simulink model "Impcont_foot_test2"  (R2016a)
settings: Solver=ode23tb  StartTime=0.0  StopTime=ti(end)  MaxStep=1e-3
InitFcn:
  | fp_sp_k = 12e3;
  | fp_sp_d = 1;
  | weights = 70/6;
  | joint_k = 0*180/pi;
  | joint_d = 0*180/pi;
  | fp_uj_dp_k = 500*180/pi;
  | fp_uj_dp_d = 1*180/pi;
  | fp_uj_ie_k = 500*180/pi;
  | fp_uj_ie_d = 1*180/pi;
  | 
  | x_k = 0*180/pi; x_d = 0*180/pi;
  | y_k = 0*180/pi; y_d = 0*180/pi;
  | z_k = 0*180/pi; z_d = 0*180/pi;
  | 
  | %{
  | stiff_dp=0.1*180/pi; stiff_ie=1*180/pi;
  | damp_dp=1*180/pi; damp_ie=1*180/pi;
  | % offset of prosthesis from centre of FP (XZY)
  |  sta=[-0.5345-6.54e-2 0.03779 0];
  | %}
  | 
  | % initpos = inv(jacob_gaitEmul(zeros(6,1)))*[ankle.trans(1,:).'; zeros(3,1)];
  | 
  | % sta = -[initpos(1) initpos(2) initpos(3)];
StopFcn:
  | %{
  | ankle = struct('ang_dp', angle_dp_out.signals.values,'ang_ie', angle_ie_out.signals.values,...
  |            'vel_dp',vel_dp.signals.values,'vel_ie',vel_ie.signals.values,...
  |            'acc_dp',acc_dp.signals.values,'acc_ie',acc_ie.signals.values,...
  |            'trans',ankle_trans_out.signals.values);
  | shin = struct('trans', trans_shin.signals.values, 'quat', quat_shin.signals.values);
  | foot = struct('trans', trans_foot.signals.values, 'quat', quat_foot.signals.values,...
  |     'acc',acc_foot.signals.values);
  | fplate = struct('trans', trans_fp.signals.values, 'quat', quat_fp.signals.values,...
  |     'torques', fp_torque_out.signals.values, 'forces', fp_force_out.signals.values);
  | 
  | [~, ~, ankle_ej.trans, ~] = est_joint(shin, foot);
  | 
  | fpForce = quatrotate(quatinv(fplate.quat), fplate.forces);
  | fpTorque = quatrotate(quatinv(fplate.quat), fplate.torques);
  | 
  | torque = cross(fplate.trans - ankle_ej.trans, fpForce) + fpTorque;
  | 
  | regMdl_dp = regress(torque(:,3),[ankle.ang_dp ankle.vel_dp foot.acc(:,3)]);
  | regMdl_ie = regress(torque(:,1),[ankle.ang_ie ankle.vel_ie foot.acc(:,1)]);
  | analysis_si = struct('kdp',regMdl_dp(1),'bdp',regMdl_dp(2),...
  |     'kie',regMdl_ie(1),'bie',regMdl_ie(2),'Jdp',regMdl_dp(3),...
  |     'Jie',regMdl_ie(3));
  | 
  | % %{
  | regMdl_dp = regress(torque(:,3),[ankle.ang_dp ankle.vel_dp ankle.acc_dp]);
  | regMdl_ie = regress(torque(:,1),[ankle.ang_ie ankle.vel_ie ankle.acc_ie]);
  | analysis_si2 = struct('kdp',regMdl_dp(1),'bdp',regMdl_dp(2),...
  |     'kie',regMdl_ie(1),'bie',regMdl_ie(2),'Jdp',regMdl_dp(3),...
  |     'Jie',regMdl_ie(3));
  | % %}
  | 
  | % %{
  | regMdl_dp = regress(tt_dp.signals.values(:,3),[ankle.ang_dp ankle.vel_dp ankle.acc_dp]);
  | regMdl_ie = regress(tt_ie.signals.values(:,3),[ankle.ang_ie ankle.vel_ie ankle.acc_ie]);
  | analysis_si3 = struct('kdp',regMdl_dp(1),'bdp',regMdl_dp(2),...
  |     'kie',regMdl_ie(1),'bie',regMdl_ie(2),'Jdp',regMdl_dp(3),...
  |     'Jie',regMdl_ie(3));
  | % %}
  | 
  | % %{
  | regMdl_dp = regress(tt_dp.signals.values(:,3),[ankle.ang_dp ankle.vel_dp foot.acc(:,3)]);
  | regMdl_ie = regress(tt_ie.signals.values(:,3),[ankle.ang_ie ankle.vel_ie foot.acc(:,1)]);
  | analysis_si4 = struct('kdp',regMdl_dp(1),'bdp',regMdl_dp(2),...
  |     'kie',regMdl_ie(1),'bie',regMdl_ie(2),'Jdp',regMdl_dp(3),...
  |     'Jie',regMdl_ie(3));
  | % %}
  | 
  | regMdl_dp = regress(torque(:,3),[ankle.ang_dp ankle.vel_dp]);
  | regMdl_ie = regress(torque(:,1),[ankle.ang_ie ankle.vel_ie]);
  | analysis_si5 = struct('kdp',regMdl_dp(1),'bdp',regMdl_dp(2),...
  |     'kie',regMdl_ie(1),'bie',regMdl_ie(2));
  | 
  | %}
values from neighbouring files (symbols this model uses):
  N = length(shin_angles_in.signals.values)    [GaitEmu_code.m]    (also in dy1.m; dy2.m; est_joint.m = size( [body1.trans body2.trans], 1 ); impcont.m)
  s = [-atan((t2.*3.379e-4+t3+t4.*t5.*4.401e-2)./(t4.*cos(q2)));-asin(t2.*1.4870979e-5+t3.*4.401e-2-t4.*t5)]    [FK_af.m]    (also in FK_footimp.m = [atan((ree2_1.*t2.*4.401e-2+ree2_2.*t4+ree2_3.*t3+t5.*t7.*4.; FK_gaitEmul.m = [q1+t2.*t4.*4.234e-1+t3.*t5.*1.5e-3-t2.*t6.*t7.*1.5e-3-5.347; ik.m = [x; y; z]; ik_af.m = FK_af(q))
  Y = -( reshape( body1.trans', [], 1 ) - reshape( body2.trans', [], 1 ) )    [creat_joint.m]    (also in est_joint.m = -( reshape( body1.trans', [3*N 1] ) - reshape( body2.trans',)
undefined symbols (not defined in the file or in its folder): X, Z
libraries: sm_lib x274, nesl_utility x97, simulink x3, dspstat3 x2, aerolibtransform2 x1
(part 7 of 7)

== system Impcont_foot_test2/Gait Emulator/prismatic frame1/y_bar_w_weightWalk_Sim1_1_RIGID/weight_4_RIGID ==
  ReferenceFrame : sm_lib/Frames and Transforms/Reference Frame
  Solid : sm_lib/Body Elements/Solid  InertiaType=Custom  Mass=weights  MassUnits=kg  CenterOfMass=[-0.093540130299891208 0.042272178743630776 0.014999999999999999]  CenterOfMassUnits=m  MomentsOfInertia=[0.0088271162208858108 0.0088271162208858108 0.017393538113134353]  MomentsOfInertiaUnits=kg*m^2  ProductsOfInertia=[0 0 0]  ProductsOfInertiaUnits=kg*m^2  DensityBased=on  Density=1000  DensityUnits=kg/(m^3)  DoExposeReferenceFrame=on  SerializedFrames=<Frames/>  GraphicType=FromGeometry  MarkerShape=Sphere  MarkerSize=10  MarkerSizeUnits=m  GraphicVisPropType=SimpleVisualProperties  GraphicDiffuseColor=[0.792156862745098 0.81960784313725488 0.93333333333333335]  GraphicSpecularColor=[0.5 0.5 0.5 1.0]  GraphicAmbientColor=[0.15 0.15 0.15 1.0]  GraphicEmissiveColor=[0.0 0.0 0.0 1.0]  GraphicShininess=75  GraphicOpacity=1  GeometryShape=FromFile  RectangleSize=[1 1]  RectangleSizeUnits=m  BrickDimensions=[1 1 1]  BrickDimensionUnits=m  CylinderRadius=1  CylinderRadiusUnits=m  CylinderLength=1  CylinderLengthUnits=m  SphereRadius=1  SphereRadiusUnits=m  EllipsoidRadii=[1 1 1]  EllipsoidRadiiUnits=m  ExtrusionCrossSection=[1 1; -1 1; -1 -1; 1 -1]  ExtrusionCrossSectionUnits=m  ExtrusionLength=1  ExtrusionLengthUnits=m  PolygonNumSides=3  PolygonOuterRadius=1  PolygonOuterRadiusUnits=m  ExtGeomFileType=STL  ExtGeomFileName=weight_Default_sldprt.STL  ExtGeomFileUnits=m  RevolutionCrossSection=[1 1; 1 -1; 2 -1; 2 1]  RevolutionCrossSectionUnits=m  RevolutionExtent=Full  RevolutionAngle=180  RevolutionAngleUnits=deg
  F : PMIOPort  Port=1  Side=Left
  connections:
  Solid/RConn1 -- ReferenceFrame/RConn1 -- F/RConn1

== system Impcont_foot_test2/Gait Emulator/prismatic frame1/y_bar_w_weightWalk_Sim1_1_RIGID/weight_5_RIGID ==
  ReferenceFrame : sm_lib/Frames and Transforms/Reference Frame
  Solid : sm_lib/Body Elements/Solid  InertiaType=Custom  Mass=weights  MassUnits=kg  CenterOfMass=[-0.093540130299891208 0.042272178743630776 0.014999999999999999]  CenterOfMassUnits=m  MomentsOfInertia=[0.0088271162208858108 0.0088271162208858108 0.017393538113134353]  MomentsOfInertiaUnits=kg*m^2  ProductsOfInertia=[0 0 0]  ProductsOfInertiaUnits=kg*m^2  DensityBased=on  Density=1000  DensityUnits=kg/(m^3)  DoExposeReferenceFrame=on  SerializedFrames=<Frames/>  GraphicType=FromGeometry  MarkerShape=Sphere  MarkerSize=10  MarkerSizeUnits=m  GraphicVisPropType=SimpleVisualProperties  GraphicDiffuseColor=[0.792156862745098 0.81960784313725488 0.93333333333333335]  GraphicSpecularColor=[0.5 0.5 0.5 1.0]  GraphicAmbientColor=[0.15 0.15 0.15 1.0]  GraphicEmissiveColor=[0.0 0.0 0.0 1.0]  GraphicShininess=75  GraphicOpacity=1  GeometryShape=FromFile  RectangleSize=[1 1]  RectangleSizeUnits=m  BrickDimensions=[1 1 1]  BrickDimensionUnits=m  CylinderRadius=1  CylinderRadiusUnits=m  CylinderLength=1  CylinderLengthUnits=m  SphereRadius=1  SphereRadiusUnits=m  EllipsoidRadii=[1 1 1]  EllipsoidRadiiUnits=m  ExtrusionCrossSection=[1 1; -1 1; -1 -1; 1 -1]  ExtrusionCrossSectionUnits=m  ExtrusionLength=1  ExtrusionLengthUnits=m  PolygonNumSides=3  PolygonOuterRadius=1  PolygonOuterRadiusUnits=m  ExtGeomFileType=STL  ExtGeomFileName=weight_Default_sldprt.STL  ExtGeomFileUnits=m  RevolutionCrossSection=[1 1; 1 -1; 2 -1; 2 1]  RevolutionCrossSectionUnits=m  RevolutionExtent=Full  RevolutionAngle=180  RevolutionAngleUnits=deg
  F : PMIOPort  Port=1  Side=Left
  connections:
  Solid/RConn1 -- ReferenceFrame/RConn1 -- F/RConn1

== system Impcont_foot_test2/Gait Emulator/prismatic frame1/y_bar_w_weightWalk_Sim1_1_RIGID/weight_6_RIGID ==
  ReferenceFrame : sm_lib/Frames and Transforms/Reference Frame
  Solid : sm_lib/Body Elements/Solid  InertiaType=Custom  Mass=weights  MassUnits=kg  CenterOfMass=[-0.093540130299891208 0.042272178743630776 0.014999999999999999]  CenterOfMassUnits=m  MomentsOfInertia=[0.0088271162208858108 0.0088271162208858108 0.017393538113134353]  MomentsOfInertiaUnits=kg*m^2  ProductsOfInertia=[0 0 0]  ProductsOfInertiaUnits=kg*m^2  DensityBased=on  Density=1000  DensityUnits=kg/(m^3)  DoExposeReferenceFrame=on  SerializedFrames=<Frames/>  GraphicType=FromGeometry  MarkerShape=Sphere  MarkerSize=10  MarkerSizeUnits=m  GraphicVisPropType=SimpleVisualProperties  GraphicDiffuseColor=[0.792156862745098 0.81960784313725488 0.93333333333333335]  GraphicSpecularColor=[0.5 0.5 0.5 1.0]  GraphicAmbientColor=[0.15 0.15 0.15 1.0]  GraphicEmissiveColor=[0.0 0.0 0.0 1.0]  GraphicShininess=75  GraphicOpacity=1  GeometryShape=FromFile  RectangleSize=[1 1]  RectangleSizeUnits=m  BrickDimensions=[1 1 1]  BrickDimensionUnits=m  CylinderRadius=1  CylinderRadiusUnits=m  CylinderLength=1  CylinderLengthUnits=m  SphereRadius=1  SphereRadiusUnits=m  EllipsoidRadii=[1 1 1]  EllipsoidRadiiUnits=m  ExtrusionCrossSection=[1 1; -1 1; -1 -1; 1 -1]  ExtrusionCrossSectionUnits=m  ExtrusionLength=1  ExtrusionLengthUnits=m  PolygonNumSides=3  PolygonOuterRadius=1  PolygonOuterRadiusUnits=m  ExtGeomFileType=STL  ExtGeomFileName=weight_Default_sldprt.STL  ExtGeomFileUnits=m  RevolutionCrossSection=[1 1; 1 -1; 2 -1; 2 1]  RevolutionCrossSectionUnits=m  RevolutionExtent=Full  RevolutionAngle=180  RevolutionAngleUnits=deg
  F : PMIOPort  Port=1  Side=Left
  connections:
  Solid/RConn1 -- ReferenceFrame/RConn1 -- F/RConn1

== system Impcont_foot_test2/Gait Emulator/prismatic frame1/y_bar_w_weightWalk_Sim1_1_RIGID/y_bar_1_RIGID ==
  ReferenceFrame : sm_lib/Frames and Transforms/Reference Frame
  Solid : sm_lib/Body Elements/Solid  InertiaType=Custom  Mass=1.29  MassUnits=kg  CenterOfMass=[0.00076616175672379865 -0.25377093214757318 3.5664030409292288e-05]  CenterOfMassUnits=m  MomentsOfInertia=[0.010298158029361381 7.4602586681976561e-05 0.010304194450422657]*(0.1/0.47799554976271263)  MomentsOfInertiaUnits=kg*m^2  ProductsOfInertia=[-6.4284014840620861e-08 -2.8526588755049515e-07 -1.380997973988322e-06]*(0.1/0.47799554976271263)  ProductsOfInertiaUnits=kg*m^2  DensityBased=on  Density=1000  DensityUnits=kg/(m^3)  DoExposeReferenceFrame=on  SerializedFrames=<Frames/>  GraphicType=FromGeometry  MarkerShape=Sphere  MarkerSize=10  MarkerSizeUnits=m  GraphicVisPropType=SimpleVisualProperties  GraphicDiffuseColor=[1.0 0.0 0.2]  GraphicSpecularColor=[0.5 0.5 0.5 1.0]  GraphicAmbientColor=[0.15 0.15 0.15 1.0]  GraphicEmissiveColor=[0.0 0.0 0.0 1.0]  GraphicShininess=75  GraphicOpacity=1  GeometryShape=FromFile  RectangleSize=[1 1]  RectangleSizeUnits=m  BrickDimensions=[1 1 1]  BrickDimensionUnits=m  CylinderRadius=1  CylinderRadiusUnits=m  CylinderLength=1  CylinderLengthUnits=m  SphereRadius=1  SphereRadiusUnits=m  EllipsoidRadii=[1 1 1]  EllipsoidRadiiUnits=m  ExtrusionCrossSection=[1 1; -1 1; -1 -1; 1 -1]  ExtrusionCrossSectionUnits=m  ExtrusionLength=1  ExtrusionLengthUnits=m  PolygonNumSides=3  PolygonOuterRadius=1  PolygonOuterRadiusUnits=m  ExtGeomFileType=STL  ExtGeomFileName=y_bar_Default_sldprt.STL  ExtGeomFileUnits=m  RevolutionCrossSection=[1 1; 1 -1; 2 -1; 2 1]  RevolutionCrossSectionUnits=m  RevolutionExtent=Full  RevolutionAngle=180  RevolutionAngleUnits=deg
  F : PMIOPort  Port=1  Side=Left
  connections:
  Solid/RConn1 -- ReferenceFrame/RConn1 -- F/RConn1

== system Impcont_foot_test2/Gait Emulator/Walkway & force plate/Force Plate/base_frame_1_RIGID/x8020_1020_1020_X_50cm_1_RIGID ==
  ReferenceFrame : sm_lib/Frames and Transforms/Reference Frame
  Solid : sm_lib/Body Elements/Solid  InertiaType=Custom  Mass=0.25907382645160842  MassUnits=kg  CenterOfMass=[0 0 0]  CenterOfMassUnits=in  MomentsOfInertia=[8.3933307234335093 8.4665424365077708 0.12805533197749852]  MomentsOfInertiaUnits=kg*in^2  ProductsOfInertia=[0 0 0]  ProductsOfInertiaUnits=kg*in^2  DensityBased=on  Density=1000  DensityUnits=kg/(m^3)  DoExposeReferenceFrame=on  SerializedFrames=<Frames/>  GraphicType=FromGeometry  MarkerShape=Sphere  MarkerSize=10  MarkerSizeUnits=m  GraphicVisPropType=SimpleVisualProperties  GraphicDiffuseColor=[1 1 1]  GraphicSpecularColor=[0.5 0.5 0.5 1.0]  GraphicAmbientColor=[0.15 0.15 0.15 1.0]  GraphicEmissiveColor=[0.0 0.0 0.0 1.0]  GraphicShininess=75  GraphicOpacity=1  GeometryShape=FromFile  RectangleSize=[1 1]  RectangleSizeUnits=m  BrickDimensions=[1 1 1]  BrickDimensionUnits=m  CylinderRadius=1  CylinderRadiusUnits=m  CylinderLength=1  CylinderLengthUnits=m  SphereRadius=1  SphereRadiusUnits=m  EllipsoidRadii=[1 1 1]  EllipsoidRadiiUnits=m  ExtrusionCrossSection=[1 1; -1 1; -1 -1; 1 -1]  ExtrusionCrossSectionUnits=m  ExtrusionLength=1  ExtrusionLengthUnits=m  PolygonNumSides=3  PolygonOuterRadius=1  PolygonOuterRadiusUnits=m  ExtGeomFileType=STL  ExtGeomFileName=8020-1020-1020 X 50cm_Default_sldprt.STL  ExtGeomFileUnits=in  RevolutionCrossSection=[1 1; 1 -1; 2 -1; 2 1]  RevolutionCrossSectionUnits=m  RevolutionExtent=Full  RevolutionAngle=180  RevolutionAngleUnits=deg
  F : PMIOPort  Port=1  Side=Left
  connections:
  ReferenceFrame/RConn1 -- Solid/RConn1 -- F/RConn1

== system Impcont_foot_test2/Gait Emulator/Walkway & force plate/Force Plate/base_frame_1_RIGID/x8020_1020_1020_X_50cm_2_RIGID ==
  ReferenceFrame : sm_lib/Frames and Transforms/Reference Frame
  Solid : sm_lib/Body Elements/Solid  InertiaType=Custom  Mass=0.25907382645160842  MassUnits=kg  CenterOfMass=[0 0 0]  CenterOfMassUnits=in  MomentsOfInertia=[8.3933307234335093 8.4665424365077708 0.12805533197749852]  MomentsOfInertiaUnits=kg*in^2  ProductsOfInertia=[0 0 0]  ProductsOfInertiaUnits=kg*in^2  DensityBased=on  Density=1000  DensityUnits=kg/(m^3)  DoExposeReferenceFrame=on  SerializedFrames=<Frames/>  GraphicType=FromGeometry  MarkerShape=Sphere  MarkerSize=10  MarkerSizeUnits=m  GraphicVisPropType=SimpleVisualProperties  GraphicDiffuseColor=[1 1 1]  GraphicSpecularColor=[0.5 0.5 0.5 1.0]  GraphicAmbientColor=[0.15 0.15 0.15 1.0]  GraphicEmissiveColor=[0.0 0.0 0.0 1.0]  GraphicShininess=75  GraphicOpacity=1  GeometryShape=FromFile  RectangleSize=[1 1]  RectangleSizeUnits=m  BrickDimensions=[1 1 1]  BrickDimensionUnits=m  CylinderRadius=1  CylinderRadiusUnits=m  CylinderLength=1  CylinderLengthUnits=m  SphereRadius=1  SphereRadiusUnits=m  EllipsoidRadii=[1 1 1]  EllipsoidRadiiUnits=m  ExtrusionCrossSection=[1 1; -1 1; -1 -1; 1 -1]  ExtrusionCrossSectionUnits=m  ExtrusionLength=1  ExtrusionLengthUnits=m  PolygonNumSides=3  PolygonOuterRadius=1  PolygonOuterRadiusUnits=m  ExtGeomFileType=STL  ExtGeomFileName=8020-1020-1020 X 50cm_Default_sldprt.STL  ExtGeomFileUnits=in  RevolutionCrossSection=[1 1; 1 -1; 2 -1; 2 1]  RevolutionCrossSectionUnits=m  RevolutionExtent=Full  RevolutionAngle=180  RevolutionAngleUnits=deg
  F : PMIOPort  Port=1  Side=Left
  connections:
  ReferenceFrame/RConn1 -- Solid/RConn1 -- F/RConn1

== system Impcont_foot_test2/Gait Emulator/Walkway & force plate/Force Plate/base_frame_1_RIGID/x8020_1020_1020_X_7_81_1_RIGID ==
  ReferenceFrame : sm_lib/Frames and Transforms/Reference Frame
  Solid : sm_lib/Body Elements/Solid  InertiaType=Custom  Mass=0.10278722807147889  MassUnits=kg  CenterOfMass=[0 0 0]  CenterOfMassUnits=in  MomentsOfInertia=[0.53334790666301179 0.56239456549511713 0.050805798463005557]  MomentsOfInertiaUnits=kg*in^2  ProductsOfInertia=[0 0 0]  ProductsOfInertiaUnits=kg*in^2  DensityBased=on  Density=1000  DensityUnits=kg/(m^3)  DoExposeReferenceFrame=on  SerializedFrames=<Frames/>  GraphicType=FromGeometry  MarkerShape=Sphere  MarkerSize=10  MarkerSizeUnits=m  GraphicVisPropType=SimpleVisualProperties  GraphicDiffuseColor=[1 1 1]  GraphicSpecularColor=[0.5 0.5 0.5 1.0]  GraphicAmbientColor=[0.15 0.15 0.15 1.0]  GraphicEmissiveColor=[0.0 0.0 0.0 1.0]  GraphicShininess=75  GraphicOpacity=1  GeometryShape=FromFile  RectangleSize=[1 1]  RectangleSizeUnits=m  BrickDimensions=[1 1 1]  BrickDimensionUnits=m  CylinderRadius=1  CylinderRadiusUnits=m  CylinderLength=1  CylinderLengthUnits=m  SphereRadius=1  SphereRadiusUnits=m  EllipsoidRadii=[1 1 1]  EllipsoidRadiiUnits=m  ExtrusionCrossSection=[1 1; -1 1; -1 -1; 1 -1]  ExtrusionCrossSectionUnits=m  ExtrusionLength=1  ExtrusionLengthUnits=m  PolygonNumSides=3  PolygonOuterRadius=1  PolygonOuterRadiusUnits=m  ExtGeomFileType=STL  ExtGeomFileName=8020-1020-1020 X 7_81_Default_sldprt.STL  ExtGeomFileUnits=in  RevolutionCrossSection=[1 1; 1 -1; 2 -1; 2 1]  RevolutionCrossSectionUnits=m  RevolutionExtent=Full  RevolutionAngle=180  RevolutionAngleUnits=deg
  F : PMIOPort  Port=1  Side=Left
  connections:
  ReferenceFrame/RConn1 -- Solid/RConn1 -- F/RConn1

== system Impcont_foot_test2/Gait Emulator/Walkway & force plate/Force Plate/base_frame_1_RIGID/x8020_1020_1020_X_7_81_2_RIGID ==
  ReferenceFrame : sm_lib/Frames and Transforms/Reference Frame
  Solid : sm_lib/Body Elements/Solid  InertiaType=Custom  Mass=0.10278722807147889  MassUnits=kg  CenterOfMass=[0 0 0]  CenterOfMassUnits=in  MomentsOfInertia=[0.53334790666301179 0.56239456549511713 0.050805798463005557]  MomentsOfInertiaUnits=kg*in^2  ProductsOfInertia=[0 0 0]  ProductsOfInertiaUnits=kg*in^2  DensityBased=on  Density=1000  DensityUnits=kg/(m^3)  DoExposeReferenceFrame=on  SerializedFrames=<Frames/>  GraphicType=FromGeometry  MarkerShape=Sphere  MarkerSize=10  MarkerSizeUnits=m  GraphicVisPropType=SimpleVisualProperties  GraphicDiffuseColor=[1 1 1]  GraphicSpecularColor=[0.5 0.5 0.5 1.0]  GraphicAmbientColor=[0.15 0.15 0.15 1.0]  GraphicEmissiveColor=[0.0 0.0 0.0 1.0]  GraphicShininess=75  GraphicOpacity=1  GeometryShape=FromFile  RectangleSize=[1 1]  RectangleSizeUnits=m  BrickDimensions=[1 1 1]  BrickDimensionUnits=m  CylinderRadius=1  CylinderRadiusUnits=m  CylinderLength=1  CylinderLengthUnits=m  SphereRadius=1  SphereRadiusUnits=m  EllipsoidRadii=[1 1 1]  EllipsoidRadiiUnits=m  ExtrusionCrossSection=[1 1; -1 1; -1 -1; 1 -1]  ExtrusionCrossSectionUnits=m  ExtrusionLength=1  ExtrusionLengthUnits=m  PolygonNumSides=3  PolygonOuterRadius=1  PolygonOuterRadiusUnits=m  ExtGeomFileType=STL  ExtGeomFileName=8020-1020-1020 X 7_81_Default_sldprt.STL  ExtGeomFileUnits=in  RevolutionCrossSection=[1 1; 1 -1; 2 -1; 2 1]  RevolutionCrossSectionUnits=m  RevolutionExtent=Full  RevolutionAngle=180  RevolutionAngleUnits=deg
  F : PMIOPort  Port=1  Side=Left
  connections:
  ReferenceFrame/RConn1 -- Solid/RConn1 -- F/RConn1

== system Impcont_foot_test2/Gait Emulator/Walkway & force plate/Force Plate/base_frame_1_RIGID/x8020_1020_1020_X_7_81_3_RIGID ==
  ReferenceFrame : sm_lib/Frames and Transforms/Reference Frame
  Solid : sm_lib/Body Elements/Solid  InertiaType=Custom  Mass=0.10278722807147889  MassUnits=kg  CenterOfMass=[0 0 0]  CenterOfMassUnits=in  MomentsOfInertia=[0.53334790666301179 0.56239456549511713 0.050805798463005557]  MomentsOfInertiaUnits=kg*in^2  ProductsOfInertia=[0 0 0]  ProductsOfInertiaUnits=kg*in^2  DensityBased=on  Density=1000  DensityUnits=kg/(m^3)  DoExposeReferenceFrame=on  SerializedFrames=<Frames/>  GraphicType=FromGeometry  MarkerShape=Sphere  MarkerSize=10  MarkerSizeUnits=m  GraphicVisPropType=SimpleVisualProperties  GraphicDiffuseColor=[1 1 1]  GraphicSpecularColor=[0.5 0.5 0.5 1.0]  GraphicAmbientColor=[0.15 0.15 0.15 1.0]  GraphicEmissiveColor=[0.0 0.0 0.0 1.0]  GraphicShininess=75  GraphicOpacity=1  GeometryShape=FromFile  RectangleSize=[1 1]  RectangleSizeUnits=m  BrickDimensions=[1 1 1]  BrickDimensionUnits=m  CylinderRadius=1  CylinderRadiusUnits=m  CylinderLength=1  CylinderLengthUnits=m  SphereRadius=1  SphereRadiusUnits=m  EllipsoidRadii=[1 1 1]  EllipsoidRadiiUnits=m  ExtrusionCrossSection=[1 1; -1 1; -1 -1; 1 -1]  ExtrusionCrossSectionUnits=m  ExtrusionLength=1  ExtrusionLengthUnits=m  PolygonNumSides=3  PolygonOuterRadius=1  PolygonOuterRadiusUnits=m  ExtGeomFileType=STL  ExtGeomFileName=8020-1020-1020 X 7_81_Default_sldprt.STL  ExtGeomFileUnits=in  RevolutionCrossSection=[1 1; 1 -1; 2 -1; 2 1]  RevolutionCrossSectionUnits=m  RevolutionExtent=Full  RevolutionAngle=180  RevolutionAngleUnits=deg
  F : PMIOPort  Port=1  Side=Left
  connections:
  ReferenceFrame/RConn1 -- Solid/RConn1 -- F/RConn1

== system Impcont_foot_test2/Gait Emulator/Walkway & force plate/Force Plate/top_frame_1_RIGID/frame1_1_RIGID ==
  ReferenceFrame : sm_lib/Frames and Transforms/Reference Frame
  Transform : sm_lib/Frames and Transforms/Rigid Transform  TranslationMethod=Cartesian  TranslationLengthUnit=m  TranslationStandardAxis=+Z  TranslationStandardOffset=0  TranslationCartesianOffset=[0.099187000000000025 -1.27675647831893e-15 -0.24999950000000001]  TranslationROffset=0  TranslationROffsetUnits=m  TranslationZOffset=0  TranslationZOffsetUnits=m  TranslationThetaOffset=0  TranslationThetaOffsetUnits=deg  RotationMethod=None  RotationAngleUnits=deg  RotationStandardAxis=+Z  RotationAngle=0.0  RotationArbitraryAxis=[0 0 1]  FollAlignAxisA=+X  BaseAlignAxisA=+Y  FollAlignAxisB=+Y  BaseAlignAxisB=+Z  RotationSequenceAxes=FollowerAxes  RotationSequence=XYX  RotationSequenceAngles=[0 0 0]  RotationSequenceAnglesUnits=deg  RotationMatrix=[1 0 0; 0 1 0; 0 0 1]
  Transform1 : sm_lib/Frames and Transforms/Rigid Transform  TranslationMethod=Cartesian  TranslationLengthUnit=m  TranslationStandardAxis=+Z  TranslationStandardOffset=0  TranslationCartesianOffset=[0.22377399999999997 0 -0.47459899999999999]  TranslationROffset=0  TranslationROffsetUnits=m  TranslationZOffset=0  TranslationZOffsetUnits=m  TranslationThetaOffset=0  TranslationThetaOffsetUnits=deg  RotationMethod=ArbitraryAxis  RotationAngleUnits=rad  RotationStandardAxis=+Z  RotationAngle=1.5707963267948968  RotationArbitraryAxis=[2.10991883731723e-15 1 5.8442032848726394e-16]  FollAlignAxisA=+X  BaseAlignAxisA=+Y  FollAlignAxisB=+Y  BaseAlignAxisB=+Z  RotationSequenceAxes=FollowerAxes  RotationSequence=XYX  RotationSequenceAngles=[0 0 0]  RotationSequenceAnglesUnits=deg  RotationMatrix=[1 0 0; 0 1 0; 0 0 1]
  Transform2 : sm_lib/Frames and Transforms/Rigid Transform  TranslationMethod=Cartesian  TranslationLengthUnit=m  TranslationStandardAxis=+Z  TranslationStandardOffset=0  TranslationCartesianOffset=[0.34836099999999992 -2.400857290751901e-15 -0.24999950000000001]  TranslationROffset=0  TranslationROffsetUnits=m  TranslationZOffset=0  TranslationZOffsetUnits=m  TranslationThetaOffset=0  TranslationThetaOffsetUnits=deg  RotationMethod=ArbitraryAxis  RotationAngleUnits=rad  RotationStandardAxis=+Z  RotationAngle=3.1415926535897931  RotationArbitraryAxis=[1.2403272853234171e-15 1 -5.0658111711395872e-16]  FollAlignAxisA=+X  BaseAlignAxisA=+Y  FollAlignAxisB=+Y  BaseAlignAxisB=+Z  RotationSequenceAxes=FollowerAxes  RotationSequence=XYX  RotationSequenceAngles=[0 0 0]  RotationSequenceAnglesUnits=deg  RotationMatrix=[1 0 0; 0 1 0; 0 0 1]
  Transform3 : sm_lib/Frames and Transforms/Rigid Transform  TranslationMethod=Cartesian  TranslationLengthUnit=m  TranslationStandardAxis=+Z  TranslationStandardOffset=0  TranslationCartesianOffset=[0.22377399999999986 -1.3322676295501878e-15 -0.025400000000000061]  TranslationROffset=0  TranslationROffsetUnits=m  TranslationZOffset=0  TranslationZOffsetUnits=m  TranslationThetaOffset=0  TranslationThetaOffsetUnits=deg  RotationMethod=ArbitraryAxis  RotationAngleUnits=rad  RotationStandardAxis=+Z  RotationAngle=1.5707963267948968  RotationArbitraryAxis=[-4.7691944979696082e-15 -1 -6.6899476726480988e-16]  FollAlignAxisA=+X  BaseAlignAxisA=+Y  FollAlignAxisB=+Y  BaseAlignAxisB=+Z  RotationSequenceAxes=FollowerAxes  RotationSequence=XYX  RotationSequenceAngles=[0 0 0]  RotationSequenceAnglesUnits=deg  RotationMatrix=[1 0 0; 0 1 0; 0 0 1]
  Transform4 : sm_lib/Frames and Transforms/Rigid Transform  TranslationMethod=Cartesian  TranslationLengthUnit=m  TranslationStandardAxis=+Z  TranslationStandardOffset=0  TranslationCartesianOffset=[-0.24999899999999994 0.025400000000001838 -0.22377400000000008]  TranslationROffset=0  TranslationROffsetUnits=m  TranslationZOffset=0  TranslationZOffsetUnits=m  TranslationThetaOffset=0  TranslationThetaOffsetUnits=deg  RotationMethod=ArbitraryAxis  RotationAngleUnits=rad  RotationStandardAxis=+Z  RotationAngle=1.5707963267948968  RotationArbitraryAxis=[-3.5952694497400173e-15 -1 1.7432631046654889e-15]  FollAlignAxisA=+X  BaseAlignAxisA=+Y  FollAlignAxisB=+Y  BaseAlignAxisB=+Z  RotationSequenceAxes=FollowerAxes  RotationSequence=XYX  RotationSequenceAngles=[0 0 0]  RotationSequenceAnglesUnits=deg  RotationMatrix=[1 0 0; 0 1 0; 0 0 1]
  x8020_1020_1020_X_50cm_1_RIGID : Subsystem
  x8020_1020_1020_X_50cm_2_RIGID : Subsystem
  x8020_1020_1020_X_7_81_1_RIGID : Subsystem
  x8020_1020_1020_X_7_81_2_RIGID : Subsystem
  F : PMIOPort  Port=1  Side=Right
  connections:
  Transform/RConn1 -- x8020_1020_1020_X_50cm_1_RIGID/LConn1
  Transform1/RConn1 -- x8020_1020_1020_X_7_81_1_RIGID/LConn1
  Transform2/RConn1 -- x8020_1020_1020_X_50cm_2_RIGID/LConn1
  Transform3/RConn1 -- x8020_1020_1020_X_7_81_2_RIGID/LConn1
  ReferenceFrame/RConn1 -- Transform2/LConn1 -- Transform3/LConn1 -- Transform/LConn1 -- Transform1/LConn1 -- Transform4/RConn1
  Transform4/LConn1 -- F/RConn1

== system Impcont_foot_test2/Gait Emulator/Walkway & force plate/Force Plate/top_frame_1_RIGID/x8020_1020_1020_X_11_81_1_RIGID ==
  ReferenceFrame : sm_lib/Frames and Transforms/Reference Frame
  Solid : sm_lib/Body Elements/Solid  InertiaType=Custom  Mass=0.15543113489425955  MassUnits=kg  CenterOfMass=[0 0 0]  CenterOfMassUnits=in  MomentsOfInertia=[1.8230290687756983 1.8669523774577936 0.076826693962624301]  MomentsOfInertiaUnits=kg*in^2  ProductsOfInertia=[0 0 0]  ProductsOfInertiaUnits=kg*in^2  DensityBased=on  Density=1000  DensityUnits=kg/(m^3)  DoExposeReferenceFrame=on  SerializedFrames=<Frames/>  GraphicType=FromGeometry  MarkerShape=Sphere  MarkerSize=10  MarkerSizeUnits=m  GraphicVisPropType=SimpleVisualProperties  GraphicDiffuseColor=[1 1 1]  GraphicSpecularColor=[0.5 0.5 0.5 1.0]  GraphicAmbientColor=[0.15 0.15 0.15 1.0]  GraphicEmissiveColor=[0.0 0.0 0.0 1.0]  GraphicShininess=75  GraphicOpacity=1  GeometryShape=FromFile  RectangleSize=[1 1]  RectangleSizeUnits=m  BrickDimensions=[1 1 1]  BrickDimensionUnits=m  CylinderRadius=1  CylinderRadiusUnits=m  CylinderLength=1  CylinderLengthUnits=m  SphereRadius=1  SphereRadiusUnits=m  EllipsoidRadii=[1 1 1]  EllipsoidRadiiUnits=m  ExtrusionCrossSection=[1 1; -1 1; -1 -1; 1 -1]  ExtrusionCrossSectionUnits=m  ExtrusionLength=1  ExtrusionLengthUnits=m  PolygonNumSides=3  PolygonOuterRadius=1  PolygonOuterRadiusUnits=m  ExtGeomFileType=STL  ExtGeomFileName=8020-1020-1020 X 11_81_Default_sldprt.STL  ExtGeomFileUnits=in  RevolutionCrossSection=[1 1; 1 -1; 2 -1; 2 1]  RevolutionCrossSectionUnits=m  RevolutionExtent=Full  RevolutionAngle=180  RevolutionAngleUnits=deg
  F : PMIOPort  Port=1  Side=Left
  connections:
  ReferenceFrame/RConn1 -- Solid/RConn1 -- F/RConn1

== system Impcont_foot_test2/Gait Emulator/Walkway & force plate/Force Plate/top_frame_1_RIGID/frame1_1_RIGID/x8020_1020_1020_X_50cm_1_RIGID ==
  ReferenceFrame : sm_lib/Frames and Transforms/Reference Frame
  Solid : sm_lib/Body Elements/Solid  InertiaType=Custom  Mass=0.25907382645160842  MassUnits=kg  CenterOfMass=[0 0 0]  CenterOfMassUnits=in  MomentsOfInertia=[8.3933307234335093 8.4665424365077708 0.12805533197749852]  MomentsOfInertiaUnits=kg*in^2  ProductsOfInertia=[0 0 0]  ProductsOfInertiaUnits=kg*in^2  DensityBased=on  Density=1000  DensityUnits=kg/(m^3)  DoExposeReferenceFrame=on  SerializedFrames=<Frames/>  GraphicType=FromGeometry  MarkerShape=Sphere  MarkerSize=10  MarkerSizeUnits=m  GraphicVisPropType=SimpleVisualProperties  GraphicDiffuseColor=[1 1 1]  GraphicSpecularColor=[0.5 0.5 0.5 1.0]  GraphicAmbientColor=[0.15 0.15 0.15 1.0]  GraphicEmissiveColor=[0.0 0.0 0.0 1.0]  GraphicShininess=75  GraphicOpacity=1  GeometryShape=FromFile  RectangleSize=[1 1]  RectangleSizeUnits=m  BrickDimensions=[1 1 1]  BrickDimensionUnits=m  CylinderRadius=1  CylinderRadiusUnits=m  CylinderLength=1  CylinderLengthUnits=m  SphereRadius=1  SphereRadiusUnits=m  EllipsoidRadii=[1 1 1]  EllipsoidRadiiUnits=m  ExtrusionCrossSection=[1 1; -1 1; -1 -1; 1 -1]  ExtrusionCrossSectionUnits=m  ExtrusionLength=1  ExtrusionLengthUnits=m  PolygonNumSides=3  PolygonOuterRadius=1  PolygonOuterRadiusUnits=m  ExtGeomFileType=STL  ExtGeomFileName=8020-1020-1020 X 50cm_Default_sldprt.STL  ExtGeomFileUnits=in  RevolutionCrossSection=[1 1; 1 -1; 2 -1; 2 1]  RevolutionCrossSectionUnits=m  RevolutionExtent=Full  RevolutionAngle=180  RevolutionAngleUnits=deg
  F : PMIOPort  Port=1  Side=Left
  connections:
  ReferenceFrame/RConn1 -- Solid/RConn1 -- F/RConn1

== system Impcont_foot_test2/Gait Emulator/Walkway & force plate/Force Plate/top_frame_1_RIGID/frame1_1_RIGID/x8020_1020_1020_X_50cm_2_RIGID ==
  ReferenceFrame : sm_lib/Frames and Transforms/Reference Frame
  Solid : sm_lib/Body Elements/Solid  InertiaType=Custom  Mass=0.25907382645160842  MassUnits=kg  CenterOfMass=[0 0 0]  CenterOfMassUnits=in  MomentsOfInertia=[8.3933307234335093 8.4665424365077708 0.12805533197749852]  MomentsOfInertiaUnits=kg*in^2  ProductsOfInertia=[0 0 0]  ProductsOfInertiaUnits=kg*in^2  DensityBased=on  Density=1000  DensityUnits=kg/(m^3)  DoExposeReferenceFrame=on  SerializedFrames=<Frames/>  GraphicType=FromGeometry  MarkerShape=Sphere  MarkerSize=10  MarkerSizeUnits=m  GraphicVisPropType=SimpleVisualProperties  GraphicDiffuseColor=[1 1 1]  GraphicSpecularColor=[0.5 0.5 0.5 1.0]  GraphicAmbientColor=[0.15 0.15 0.15 1.0]  GraphicEmissiveColor=[0.0 0.0 0.0 1.0]  GraphicShininess=75  GraphicOpacity=1  GeometryShape=FromFile  RectangleSize=[1 1]  RectangleSizeUnits=m  BrickDimensions=[1 1 1]  BrickDimensionUnits=m  CylinderRadius=1  CylinderRadiusUnits=m  CylinderLength=1  CylinderLengthUnits=m  SphereRadius=1  SphereRadiusUnits=m  EllipsoidRadii=[1 1 1]  EllipsoidRadiiUnits=m  ExtrusionCrossSection=[1 1; -1 1; -1 -1; 1 -1]  ExtrusionCrossSectionUnits=m  ExtrusionLength=1  ExtrusionLengthUnits=m  PolygonNumSides=3  PolygonOuterRadius=1  PolygonOuterRadiusUnits=m  ExtGeomFileType=STL  ExtGeomFileName=8020-1020-1020 X 50cm_Default_sldprt.STL  ExtGeomFileUnits=in  RevolutionCrossSection=[1 1; 1 -1; 2 -1; 2 1]  RevolutionCrossSectionUnits=m  RevolutionExtent=Full  RevolutionAngle=180  RevolutionAngleUnits=deg
  F : PMIOPort  Port=1  Side=Left
  connections:
  ReferenceFrame/RConn1 -- Solid/RConn1 -- F/RConn1

== system Impcont_foot_test2/Gait Emulator/Walkway & force plate/Force Plate/top_frame_1_RIGID/frame1_1_RIGID/x8020_1020_1020_X_7_81_1_RIGID ==
  ReferenceFrame : sm_lib/Frames and Transforms/Reference Frame
  Solid : sm_lib/Body Elements/Solid  InertiaType=Custom  Mass=0.10278722807147889  MassUnits=kg  CenterOfMass=[0 0 0]  CenterOfMassUnits=in  MomentsOfInertia=[0.53334790666301179 0.56239456549511713 0.050805798463005557]  MomentsOfInertiaUnits=kg*in^2  ProductsOfInertia=[0 0 0]  ProductsOfInertiaUnits=kg*in^2  DensityBased=on  Density=1000  DensityUnits=kg/(m^3)  DoExposeReferenceFrame=on  SerializedFrames=<Frames/>  GraphicType=FromGeometry  MarkerShape=Sphere  MarkerSize=10  MarkerSizeUnits=m  GraphicVisPropType=SimpleVisualProperties  GraphicDiffuseColor=[1 1 1]  GraphicSpecularColor=[0.5 0.5 0.5 1.0]  GraphicAmbientColor=[0.15 0.15 0.15 1.0]  GraphicEmissiveColor=[0.0 0.0 0.0 1.0]  GraphicShininess=75  GraphicOpacity=1  GeometryShape=FromFile  RectangleSize=[1 1]  RectangleSizeUnits=m  BrickDimensions=[1 1 1]  BrickDimensionUnits=m  CylinderRadius=1  CylinderRadiusUnits=m  CylinderLength=1  CylinderLengthUnits=m  SphereRadius=1  SphereRadiusUnits=m  EllipsoidRadii=[1 1 1]  EllipsoidRadiiUnits=m  ExtrusionCrossSection=[1 1; -1 1; -1 -1; 1 -1]  ExtrusionCrossSectionUnits=m  ExtrusionLength=1  ExtrusionLengthUnits=m  PolygonNumSides=3  PolygonOuterRadius=1  PolygonOuterRadiusUnits=m  ExtGeomFileType=STL  ExtGeomFileName=8020-1020-1020 X 7_81_Default_sldprt.STL  ExtGeomFileUnits=in  RevolutionCrossSection=[1 1; 1 -1; 2 -1; 2 1]  RevolutionCrossSectionUnits=m  RevolutionExtent=Full  RevolutionAngle=180  RevolutionAngleUnits=deg
  F : PMIOPort  Port=1  Side=Left
  connections:
  ReferenceFrame/RConn1 -- Solid/RConn1 -- F/RConn1

== system Impcont_foot_test2/Gait Emulator/Walkway & force plate/Force Plate/top_frame_1_RIGID/frame1_1_RIGID/x8020_1020_1020_X_7_81_2_RIGID ==
  ReferenceFrame : sm_lib/Frames and Transforms/Reference Frame
  Solid : sm_lib/Body Elements/Solid  InertiaType=Custom  Mass=0.10278722807147889  MassUnits=kg  CenterOfMass=[0 0 0]  CenterOfMassUnits=in  MomentsOfInertia=[0.53334790666301179 0.56239456549511713 0.050805798463005557]  MomentsOfInertiaUnits=kg*in^2  ProductsOfInertia=[0 0 0]  ProductsOfInertiaUnits=kg*in^2  DensityBased=on  Density=1000  DensityUnits=kg/(m^3)  DoExposeReferenceFrame=on  SerializedFrames=<Frames/>  GraphicType=FromGeometry  MarkerShape=Sphere  MarkerSize=10  MarkerSizeUnits=m  GraphicVisPropType=SimpleVisualProperties  GraphicDiffuseColor=[1 1 1]  GraphicSpecularColor=[0.5 0.5 0.5 1.0]  GraphicAmbientColor=[0.15 0.15 0.15 1.0]  GraphicEmissiveColor=[0.0 0.0 0.0 1.0]  GraphicShininess=75  GraphicOpacity=1  GeometryShape=FromFile  RectangleSize=[1 1]  RectangleSizeUnits=m  BrickDimensions=[1 1 1]  BrickDimensionUnits=m  CylinderRadius=1  CylinderRadiusUnits=m  CylinderLength=1  CylinderLengthUnits=m  SphereRadius=1  SphereRadiusUnits=m  EllipsoidRadii=[1 1 1]  EllipsoidRadiiUnits=m  ExtrusionCrossSection=[1 1; -1 1; -1 -1; 1 -1]  ExtrusionCrossSectionUnits=m  ExtrusionLength=1  ExtrusionLengthUnits=m  PolygonNumSides=3  PolygonOuterRadius=1  PolygonOuterRadiusUnits=m  ExtGeomFileType=STL  ExtGeomFileName=8020-1020-1020 X 7_81_Default_sldprt.STL  ExtGeomFileUnits=in  RevolutionCrossSection=[1 1; 1 -1; 2 -1; 2 1]  RevolutionCrossSectionUnits=m  RevolutionExtent=Full  RevolutionAngle=180  RevolutionAngleUnits=deg
  F : PMIOPort  Port=1  Side=Left
  connections:
  ReferenceFrame/RConn1 -- Solid/RConn1 -- F/RConn1

== matlab function Impcont_foot_test2/Gait Emulator/Walkway & force plate/Ground Contact/MATLAB Function ==
  data: p input; F output; v input; Q input; w input; T output; F_f output; T_f output
function [F, T, F_f, T_f] = fcn(p, v, Q, w)
%#codegen

if abs(p(1))>0.25

% R = quat2dcm(Q);
R = [1 - 2*Q(3)^2 - 2*Q(4)^2	2*Q(2)*Q(3) - 2*Q(4)*Q(1)	2*Q(2)*Q(4) + 2*Q(3)*Q(1)
     2*Q(2)*Q(3) + 2*Q(4)*Q(1)	1 - 2*Q(2)^2 - 2*Q(4)^2	2*Q(3)*Q(4) - 2*Q(2)*Q(1)
     2*Q(2)*Q(4) - 2*Q(3)*Q(1)	2*Q(3)*Q(4) + 2*Q(2)*Q(1)	1 - 2*Q(2)^2 - 2*Q(3)^2];

th1 = linspace(-pi/2,pi/2,5);
% th1 = -pi/2 : 0.7 : pi/2;
r1 = 47e-3.*[cos(th1) cos(th1); sin(th1) sin(th1); zeros(size(th1)), zeros(size(th1))]; % circle
th2 = linspace(pi/2,-pi/2,5);
% th2 = pi/2 : -0.7 : -pi/2;
r2 = 47e-3.*[-cos(th2) -cos(th2); sin(th2) sin(th2); zeros(size(th2)), zeros(size(th2))]; % circle
r1(1,:) = bsxfun(@plus,r1(1,:),134e-3/2); 
r2(1,:) = bsxfun(@minus,r2(1,:),134e-3/2);
% r = ([1 1 1; 1 1 -1; 1 -1 1; 1 -1 -1; -1 1 1; -1 1 -1; -1 -1 1; -1 -1 -1].*repmat([0.2 0.1 0],8,1).*0.5).';
% xx = linspace(-0.11,-0.03,2);

% xx = -0.07;
xx = 0;
% xx = -0.12:0.04:-0.02;
r3 = [repmat(xx,1,2);repmat(47e-3,1,length(xx)),repmat(-47e-3,1,length(xx));zeros(1,size(xx,2)*2)];
r = [r1,r2,r3,zeros(3,1)];

% spring-damper contact modelc
K = [0 0 0; 0 0 0; 0 0 10]*2e4;
B = [10 0 0; 0 10 0; 0 0 10]*2e2;
% K = [0 0 0; 0 0 0; 0 0 1]*2e3;
% B = [1 0 0; 0 1 0; 0 0 1]*2e2;

rr = bsxfun(@plus, R*r, p); % vertex position on base frame
vv = bsxfun(@plus, v, bsxfun(@cross, w, R*r)); % vertex velocity on base frame

FF = -K*(rr - 0) - B*vv; % force on vertex on base frame

% point is active if normal force is compressing ground
loss = 1 ./ ( 1 + exp(-[0 0 1]*FF) );
% loss = 1 ./ ( 1 + exp(150*[0 0 1]*rr) );

% displace force to coordinate center

% if abs(p(1))>=0.15 && abs(p(2))>=0.1
%     F=[0 0 0]';
%     T=[0 0 0]';
% else
    F = sum( repmat(loss,[3 1]) .* FF, 2 ); % contact force on base frame
    T = sum( repmat(loss,[3 1]) .* cross( R*r, FF ), 2 ); % contact torque on base frame
%     F = sum(FF, 2 ); % contact force on base frame
%     T = sum(cross( R*r, FF ), 2 ); % contact torque on base frame
    F_f = repmat(1 ./ ( 1 + exp(-[0 0 1]*FF(:,end))),[3 1]) .* FF(:,end);
    T_f = repmat(1 ./ ( 1 + exp(-[0 0 1]*FF(:,end))),[3 1]) .* cross( R*r(:,end), FF(:,end));
else
    F=[0 0 0]';
    T=[0 0 0]';
    F_f = [0 0 0]';
    T_f = [0 0 0]';
end
end

== matlab function Impcont_foot_test2/Gait Emulator/Walkway & force plate/FP Contact/MATLAB Function ==
  data: p input; F output; v input; Q input; w input; T output; F_f output; T_f output
function [F, T, F_f, T_f] = fcn(p, v, Q, w)
%#codegen

% if abs(p(1))<=0.25 && p(3)<=5e-3
if abs(p(1))<=0.25

% R = quat2dcm(Q);
R = [1 - 2*Q(3)^2 - 2*Q(4)^2	2*Q(2)*Q(3) - 2*Q(4)*Q(1)	2*Q(2)*Q(4) + 2*Q(3)*Q(1)
     2*Q(2)*Q(3) + 2*Q(4)*Q(1)	1 - 2*Q(2)^2 - 2*Q(4)^2	2*Q(3)*Q(4) - 2*Q(2)*Q(1)
     2*Q(2)*Q(4) - 2*Q(3)*Q(1)	2*Q(3)*Q(4) + 2*Q(2)*Q(1)	1 - 2*Q(2)^2 - 2*Q(3)^2];

th1 = linspace(-pi/2,pi/2,5);
% th1 = -pi/2 : 0.7 : pi/2;
r1 = 47e-3.*[cos(th1) cos(th1); sin(th1) sin(th1); zeros(size(th1)), zeros(size(th1))]; % circle
th2 = linspace(pi/2,-pi/2,5);
% th2 = pi/2 : -0.7 : -pi/2;
r2 = 47e-3.*[-cos(th2) -cos(th2); sin(th2) sin(th2); zeros(size(th2)), zeros(size(th2))]; % circle
r1(1,:) = bsxfun(@plus,r1(1,:),134e-3/2); 
r2(1,:) = bsxfun(@minus,r2(1,:),134e-3/2);
% r = ([1 1 1; 1 1 -1; 1 -1 1; 1 -1 -1; -1 1 1; -1 1 -1; -1 -1 1; -1 -1 -1].*repmat([0.2 0.1 0],8,1).*0.5).';
% xx = linspace(-0.11,-0.03,2);

% xx = -0.07;
xx = 0;
% xx = -0.12:0.04:-0.02;
r3 = [repmat(xx,1,2);repmat(47e-3,1,length(xx)),repmat(-47e-3,1,length(xx));zeros(1,size(xx,2)*2)];
r = [r1,r2,r3,zeros(3,1)];

% spring-damper contact modelc
K = [0 0 0; 0 0 0; 0 0 10]*2e4;
B = [10 0 0; 0 10 0; 0 0 10]*2e2;
% K = [0 0 0; 0 0 0; 0 0 1]*2e4;
% B = [1 0 0; 0 1 0; 0 0 1]*2e2;

rr = bsxfun(@plus, R*r, p); % vertex position on base frame
vv = bsxfun(@plus, v, bsxfun(@cross, w, R*r)); % vertex velocity on base frame

FF = -K*(rr - 0) - B*vv; % force on vertex on base frame

% point is active if normal force is compressing ground
loss = 1 ./ ( 1 + exp(-[0 0 1]*FF) );
% loss = 1 ./ ( 1 + exp(150*[0 0 1]*rr) );

% displace force to coordinate center

% if abs(p(1))>=0.15 && abs(p(2))>=0.1
%     F=[0 0 0]';
%     T=[0 0 0]';
% else
%     if any(rr(3,:)) && mean(nonzeros(rr(3,:)))<=5e-3
%     if any(rr(3,:)<=5e-5)
        F = sum( repmat(loss,[3 1]) .* FF, 2 ); % contact force on base frame
        T = sum( repmat(loss,[3 1]) .* cross( R*r, FF ), 2 ); % contact torque on base frame
%     else
%         F=[0 0 0]';
%         T=[0 0 0]';
%     end
%     F = sum(FF, 2 ); % contact force on base frame
%     T = sum(cross( R*r, FF ), 2 ); % contact torque on base frame
    F_f = repmat(1 ./ ( 1 + exp(-[0 0 1]*FF(:,end))),[3 1]) .* FF(:,end);
    T_f = repmat(1 ./ ( 1 + exp(-[0 0 1]*FF(:,end))),[3 1]) .* cross( R*r(:,end), FF(:,end));
else
    F=[0 0 0]';
    T=[0 0 0]';
    F_f = [0 0 0]';
    T_f = [0 0 0]';
end
end

== matlab function Impcont_foot_test2/MATLAB Function ==
  data: xt input; qc input; u output; qdc input; qddc input; ree input; tee input; grn_frc input; grn_trq input; quat_f input; w_f input; t_sim input
function u = roboctrl_footimp(xt,qc,qdc,qddc,ree,tee,...
    grn_frc,grn_trq,quat_f,w_f,t_sim)
%#codegen
% q is current pose of robot
% xt is target [pos vel acc]

% Mass Inertia Matrix
% mass = 83491.14e-3;
% PnI = [-2939718522.52 755286751.35 2940276623.48];
% Ixy = -254376331060.49; Iyz = -2656879652.72; Izx = 7885931500.71;
% % inertia = [PnI(1) Ixy Izx; Ixy PnI(2) Iyz; Izx Iyz PnI(3)]*1e-9;
% % [rz rx ry]
% inertia = [PnI(3) Izx Iyz; Izx PnI(1) Ixy; Iyz Ixy PnI(2)]*1e-9;
% 
% Mx = [diag(repmat(mass,1,3)) zeros(3); zeros(3) inertia];
% % Mq = [diag([0 0 mass]) zeros(3); zeros(3) inertia];
% % Mx = 1/(jacob_gaitEmul2(qc)*(massmatrix(qc)\jacob_gaitEmul2(qc).'));

% frc_ie(1) = -frc_ie(1);
% trq_ie(1) = -trq_ie(1);
% grn_trq(2) = -grn_trq(2);
% grn_frc(2) = -grn_frc(2);
% 
% % Rz = @(q) [cos(q) -sin(q) 0; sin(q) cos(q) 0; 0 0 1];
% % frc = Rz(pi) * (frc_ie([3 2 1])+frc_dp)./2;
% % trq = Rz(pi) * (trq_ie([3 2 1])+trq_dp)./2;
% frc_ie = Rz(pi) * (frc_ie([3 2 1]));
% frc_dp = Rz(pi) * (frc_dp([3 2 1]));
% trq_ie = Rz(pi) * (trq_ie([3 2 1]));
% trq_dp = Rz(pi) * (trq_dp([3 2 1]));
grn_frc = Rz(pi) * (grn_frc([3 2 1]));
grn_trq = Rz(pi) * (grn_trq([3 2 1]));

s.g = [0; -9.81; 0];
s.frc = [0 grn_frc(1); 0 grn_frc(2); 0 grn_frc(3)];
s.trq = [0 grn_trq(1); 0 grn_trq(2); 0 grn_trq(3)];
s.m = [0 1];
s.l = [0 0.0084;0 -0.0325;0 0.0254];
s.In = [0 0.0003;0 0;0 0;0 0;0 0.0011;0 0;0 0;0 0;0 0.0008];

% s.frc = [frc_ie frc_dp];
% s.trq = [trq_ie trq_dp];
% s.m = [1 1];
% s.l = [0.0084 0.0084;-0.0325 -0.0325;0.0254 0.0254];
% s.In = [0.0003 0.0003;0 0;0 0;0 0;0.0011 0.0011;0 0;0 0;0 0;0.0008 0.0008];

s.q = qc;
s.qd = qdc;
s.qdd = qddc;
[Mq,Cq] = foot_dirdyna(s);

% Gravity
% % Gq = -9.81*jacob_gaitEmul(q).'*Mq;
% W1 = 83491.14e-3;
% W2 = 4678.07e-3; %knee
% W3 = 4100e-3; %hip
% L2 = 207.58e-3;
% % Gq = [0 W1 0 L2*W2*sin(qc(4)) W3 L2*W2*sin(qc(5))].';
% Gq = [0 0 W1 L2*W2*sin(qc(4)) L2*W2*sin(qc(5)) W3].';

% Gq = -[1*-0.032495217139970998*sin(xc(1));1*-0.032495217139970998*sin(xc(2))];
% Gq = -[1*0.025447381031481243*sin(qc(1));1*0.008370045592423393*sin(qc(2))];
s.qd = zeros(2,1);
[~,Gq] = foot_dirdyna(s);

% Control Signal
% Kp = [0.1;0.1]; Kv = [1;1];
% xdes = Kp.*(xt-xc);
% xdes = Kp*(qd-qc)+Kv*(vd-vc);
% u = jacob_footimp(ree,tee,xc).'*Mq*xdes + Gq + Cq - jacob_footimp(ree,tee,xc).'*grn_trq([1 3]);
xc = quat_f([1 3]);
xdc = w_f([1 3]);

t_sta = [0.2897 0.3874 0.4851 0.5828 0.6805];
K_dp = [69.8371 113.2203 136.2177 140.6435 151.1421];
K_ie = [82.6537 80.4438 50.3841 52.903 69.9986];
B_dp = [1.1955 1.4139 1.7642 1.5009 1.2292];
B_ie = [0.5354 0.3988 0.496 0.7497 0.5964];
J_dp = [0.0196 0.033 0.0507 0.0765 0.0369];
J_ie = [0.0065 0.0058 0.0153 0.0171 0.0094];
% sl = [10.75 30.75 50.75 70.75 90.75]./100;

if mod(t_sim,3)<=t_sta(1)
    Jx = diag([J_dp(1) J_ie(1)]);
    Dx = diag([B_dp(1) B_ie(1)]);
    Kx = diag([K_dp(1) K_ie(1)]);
elseif mod(t_sim,3)<=t_sta(2)
    Jx = diag([J_dp(2) J_ie(2)]);
    Dx = diag([B_dp(2) B_ie(2)]);
    Kx = diag([K_dp(2) K_ie(2)]);
elseif mod(t_sim,3)<=t_sta(3)
    Jx = diag([J_dp(3) J_ie(3)]);
    Dx = diag([B_dp(3) B_ie(3)]);
    Kx = diag([K_dp(3) K_ie(3)]);
elseif mod(t_sim,3)<=t_sta(4)
    Jx = diag([J_dp(4) J_ie(4)]);
    Dx = diag([B_dp(4) B_ie(4)]);
    Kx = diag([K_dp(4) K_ie(4)]);
else
    Jx = diag([J_dp(5) J_ie(5)]);
    Dx = diag([B_dp(5) B_ie(5)]);
    Kx = diag([K_dp(5) K_ie(5)]);
end

% Jx = diag([0.0433 0.0108]); Dx = diag([1.4207 0.5552]); Kx = diag([122.21 67.2766]);
% Jx = diag([0.01 0.01]); Dx = diag([1e0 1e0]); Kx = diag([1e3 1e3]);
xdes = xt([5 6]) + Jx\(Dx*(xt([3 4])-xdc)+Kx*(xt([1 2])-xc)-grn_frc([1 2]));
% xdes = xt([5 6]) + Bx\(Dx*(xt([3 4])-xdc)+Kx*(xt([1 2])-xc));

% u = Mq/(jacob_footimp(ree,tee,xc))*xdes + Cq.*(jacob_footimp(ree,tee,xc)\xdc) + ...
%     Gq - jacob_footimp(ree,tee,xc).'*grn_trq([1 2]);

u = Mq/(jacob_footimp(ree,tee,qc))*xdes + Cq.*(jacob_footimp(ree,tee,qc)\xdc) + ...
    Gq - (jacob_footimp(ree,tee,qc)).'*grn_frc([1 2]);
u = Mq/(jacob_footimp(ree,tee,qc))*xdes + Cq + ...
    Gq - (jacob_footimp(ree,tee,qc)).'*grn_frc([1 2]);
% u = Mq/(jacob_footimp(ree,tee,qc))*xdes + Cq.*(jacob_footimp(ree,tee,qc)\xdc) + Gq;
end

function R = Rz(q)
    R = [cos(q) -sin(q) 0; sin(q) cos(q) 0; 0 0 1];
end

== matlab function Impcont_foot_test2/MATLAB Function2 ==
  data: t input; q input; qp output; dev output; ree input; tee input
function [qp, dev] = ik_sol_footimp(t, q ,ree, tee)
%#codegen
[qp, dev] = ik_footimp(t, q/2 ,ree, tee);

== matlab function Impcont_foot_test2/MATLAB Function1 ==
  data: t input; q input; qp output; dev output
function [qp, dev] = ik_sol(t, q)
%#codegen
[qp, dev] = ik_test(t, q/2);
